simulink model "part7_simulink"  (Simulink 7.6)
settings: Solver=ode45  StartTime=0.0  StopTime=10.0  RelTol=1e-3
libraries: simulink x2
settings Model: Creator=Docencia  LastModifiedBy=Docencia

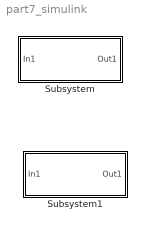
== system part7_simulink ==
  Subsystem : Subsystem
  Subsystem1 : Subsystem

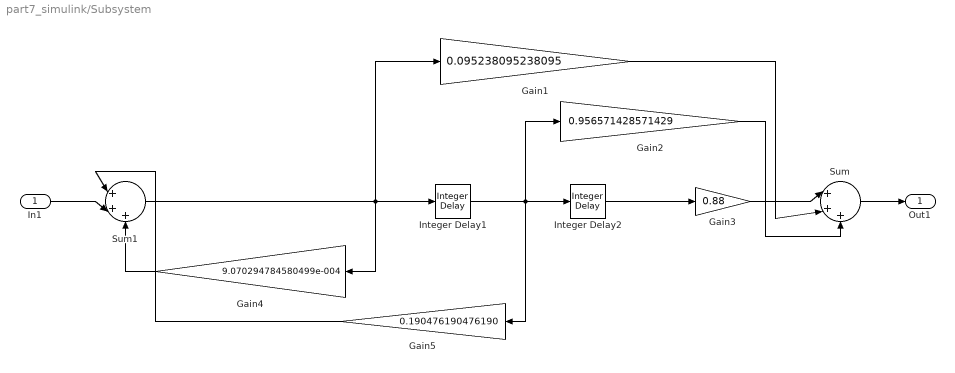
== system part7_simulink/Subsystem ==
  In1 : Inport
  Gain1 : Gain  Gain=0.095238095238095  ParamDataTypeStr=sfix(8)  OutDataTypeStr=fixdt(1,14,8)
  Gain2 : Gain  Gain=0.956571428571429  ParamDataTypeStr=sfix(8)  OutDataTypeStr=fixdt(1,14,8)
  Gain3 : Gain  Gain=0.88  ParamDataTypeStr=sfix(8)  OutDataTypeStr=fixdt(1,14,8)
  Gain4 : Gain  Gain=9.070294784580499e-004  ParamDataTypeStr=sfix(8)  OutDataTypeStr=fixdt(1,14,8)
  Gain5 : Gain  Gain=0.190476190476190  ParamDataTypeStr=sfix(8)  OutDataTypeStr=fixdt(1,14,8)
  Integer Delay1 : simulink/Discrete/Integer Delay  NumDelays=1  vinit=0.0  samptime=-1
  Integer Delay2 : simulink/Discrete/Integer Delay  NumDelays=1  vinit=0.0  samptime=-1
  Sum : Sum  Inputs=|+++
  Sum1 : Sum  Inputs=|+++
  Out1 : Outport
  wires:
  Integer Delay1/1 -> Integer Delay2/1, Gain2/1, Gain5/1
  Integer Delay2/1 -> Gain3/1
  Gain1/1 -> Sum/2
  Gain2/1 -> Sum/3
  Sum1/1 -> Integer Delay1/1, Gain4/1, Gain1/1
  Gain5/1 -> Sum1/1
  In1/1 -> Sum1/2
  Sum/1 -> Out1/1
  Gain3/1 -> Sum/1
  Gain4/1 -> Sum1/3

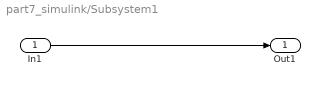
== system part7_simulink/Subsystem1 ==
  In1 : Inport
  Out1 : Outport
  wires:
  In1/1 -> Out1/1
